simulink model "blockdemo"  (Simulink 6.3)
settings: Solver=FixedStepDiscrete  StartTime=0.0  StopTime=10.0  RelTol=1e-3
InitFcn:
  | %% DSPBuilder Start
  | alt_dspbuilder_update_model(bdroot)
  | %% DSPBuilder End
libraries: allblocks_alteradspbuilder2 x14
settings Model: Creator=cpurcell  LastModifiedBy=delphick
settings DebuggingCC: MultiTaskDSMMsg=error

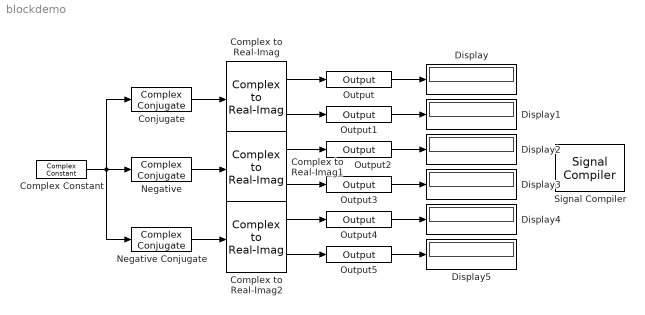
== system blockdemo ==
  Complex Constant : allblocks_alteradspbuilder2/Complex Constant  mask_cst_real=-2  mask_cst_imag=-2  BusType=Signed Integer  bwl=2  bwr=0  SpecifyClock=off
  Complex to Real-Imag : allblocks_alteradspbuilder2/Complex to Real-Imag  BusType=Signed Integer  bwl=3  bwr=0
  Complex to Real-Imag1 : allblocks_alteradspbuilder2/Complex to Real-Imag  BusType=Signed Integer  bwl=3  bwr=0
  Complex to Real-Imag2 : allblocks_alteradspbuilder2/Complex to Real-Imag  BusType=Signed Integer  bwl=3  bwr=0
  Conjugate : allblocks_alteradspbuilder2/Complex Conjugate  operation=Conjugate  register_inputs=on  use_ena=off  use_aclr=off
  Display{,1..5} (6 alike) : Display
  Negative : allblocks_alteradspbuilder2/Complex Conjugate  operation=Negative  register_inputs=on  use_ena=off  use_aclr=off
  Negative Conjugate : allblocks_alteradspbuilder2/Complex Conjugate  operation=Negative Conjugate  register_inputs=on  use_ena=off  use_aclr=off
  Output : allblocks_alteradspbuilder2/Output  iofile=C:\workspace_clean\Documentation\DesignExamples\Tutorials\UnitBlocks\Complex\ComplexConjugate\tb_blockdemo\blockdemo_Output.capture  BusType=Inferred  bwl=8  bwr=0  PORTTYPE=Output
  Output1 : allblocks_alteradspbuilder2/Output  iofile=C:\workspace_clean\Documentation\DesignExamples\Tutorials\UnitBlocks\Complex\ComplexConjugate\tb_blockdemo\blockdemo_Output1.capture  BusType=Inferred  bwl=8  bwr=0  PORTTYPE=Output
  Output2 : allblocks_alteradspbuilder2/Output  iofile=C:\workspace_clean\Documentation\DesignExamples\Tutorials\UnitBlocks\Complex\ComplexConjugate\tb_blockdemo\blockdemo_Output2.capture  BusType=Inferred  bwl=8  bwr=0  PORTTYPE=Output
  Output3 : allblocks_alteradspbuilder2/Output  iofile=C:\workspace_clean\Documentation\DesignExamples\Tutorials\UnitBlocks\Complex\ComplexConjugate\tb_blockdemo\blockdemo_Output3.capture  BusType=Inferred  bwl=8  bwr=0  PORTTYPE=Output
  Output4 : allblocks_alteradspbuilder2/Output  iofile=C:\workspace_clean\Documentation\DesignExamples\Tutorials\UnitBlocks\Complex\ComplexConjugate\tb_blockdemo\blockdemo_Output4.capture  BusType=Inferred  bwl=8  bwr=0  PORTTYPE=Output
  Output5 : allblocks_alteradspbuilder2/Output  iofile=C:\workspace_clean\Documentation\DesignExamples\Tutorials\UnitBlocks\Complex\ComplexConjugate\tb_blockdemo\blockdemo_Output5.capture  BusType=Inferred  bwl=8  bwr=0  PORTTYPE=Output
  Signal Compiler : allblocks_alteradspbuilder2/Signal Compiler  DeviceFamily=Stratix IV  DeviceName=AUTO  EnableSignalTap=off  SignalTapDepth=128  UseBoardBlock=off  StpUseDefaultClock=on  StpClock=clock
  wires:
  Complex Constant/1 -> Negative/1, Conjugate/1, Negative Conjugate/1
  Output/1 -> Display/1
  Output1/1 -> Display1/1
  Output2/1 -> Display2/1
  Output3/1 -> Display3/1
  Output4/1 -> Display4/1
  Output5/1 -> Display5/1
  Complex to Real-Imag/1 -> Output/1
  Complex to Real-Imag/2 -> Output1/1
  Complex to Real-Imag1/1 -> Output2/1
  Complex to Real-Imag1/2 -> Output3/1
  Complex to Real-Imag2/1 -> Output4/1
  Complex to Real-Imag2/2 -> Output5/1
  Conjugate/1 -> Complex to Real-Imag/1
  Negative/1 -> Complex to Real-Imag1/1
  Negative Conjugate/1 -> Complex to Real-Imag2/1
